simulink model "pack_96s"  (R2024b)
settings: Solver=ode4  StartTime=0.0  StopTime=T_stop  FixedStep=0.1  RelTol=1e-3
PreLoadFcn:
  | run(fullfile(fileparts(which('pack_96s')), '..', 'scripts', 'init_plant_model.m'));
undefined symbols (not defined in the file): cell_dSoC_pct, cell_Q_Ah, cell_RO_scale, cp_coolant, h_rad, I_bal_default, m_coolant, P_chiller_max, P_heater_max, T_cells_init, T_cool_off, T_cool_on, T_cool_target, T_heat_off, T_heat_on, T_heat_target, tau_chiller, tau_heater
settings Model: Creator=rayen  LastModifiedBy=dhia
settings DebuggingCC: AlgebraicLoopMsg=none

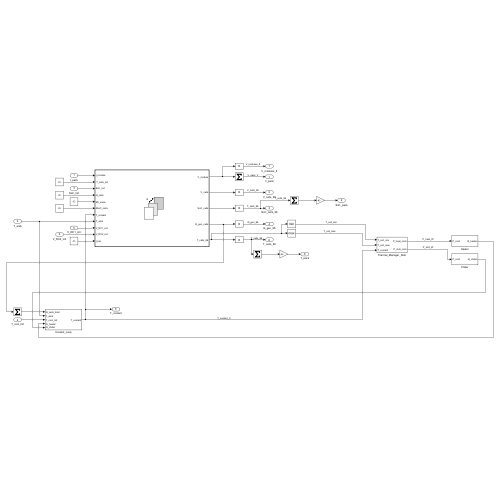
[thumbnail: Simulink's stored preview of the top-level diagram]
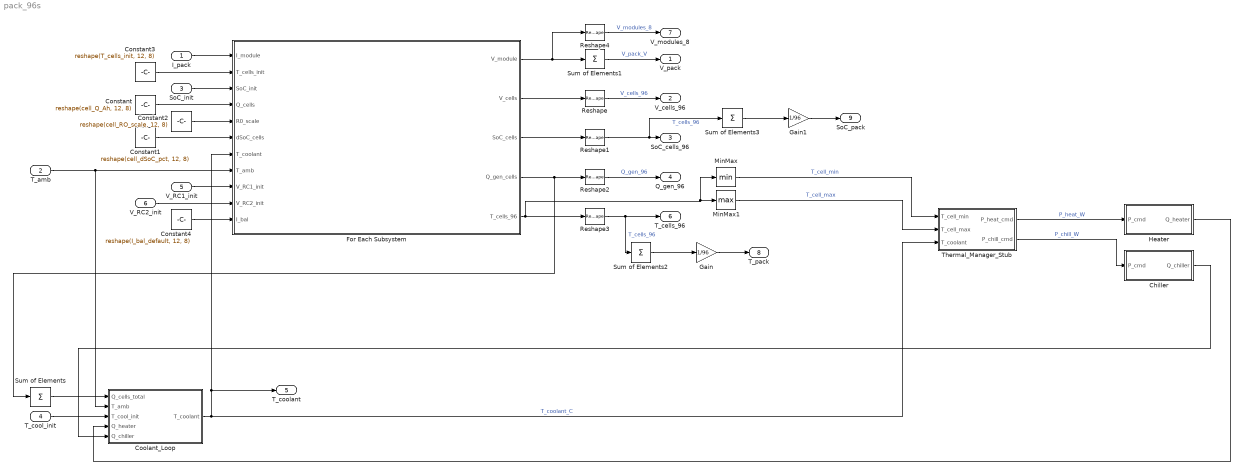
== system pack_96s ==
  I_pack : Inport
  T_amb : Inport  Port=2
  SoC_init : Inport  Port=3
  T_cool_init : Inport  Port=4
  V_RC1_init : Inport  Port=5
  V_RC2_init : Inport  Port=6
  Chiller : Subsystem
  Constant : Constant  Value=reshape(cell_Q_Ah, 12, 8)
  Constant1 : Constant  Value=reshape(cell_dSoC_pct, 12, 8)
  Constant2 : Constant  Value=reshape(cell_RO_scale, 12, 8)
  Constant3 : Constant  Value=reshape(T_cells_init, 12, 8)
  Constant4 : Constant  Value=reshape(I_bal_default, 12, 8)
  Coolant_Loop : Subsystem
  For Each Subsystem : Subsystem  TreatAsAtomicUnit=on
  Gain : Gain  Gain=1/96
  Gain1 : Gain  Gain=1/96
  Heater : Subsystem
  MinMax : MinMax
  MinMax1 : MinMax  Function=max
  Reshape{,1..3} (4 alike) : Reshape  OutputDimensionality=Customize  OutputDimensions=[96, 1]
  Reshape4 : Reshape  OutputDimensionality=Customize  OutputDimensions=[8, 1]
  Sum of Elements{,1..3} (4 alike) : Sum  Inputs=+
  Thermal_Manager_Stub : Subsystem
  V_pack : Outport
  V_cells_96 : Outport  Port=2
  SoC_cells_96 : Outport  Port=3
  Q_gen_96 : Outport  Port=4
  T_coolant : Outport  Port=5
  T_cells_96 : Outport  Port=6
  V_modules_8 : Outport  Port=7
  T_pack : Outport  Port=8
  SoC_pack : Outport  Port=9
  wires:
  I_pack/1 -> For Each Subsystem/1(I_module)
  SoC_init/1 -> For Each Subsystem/3(SoC_init)
  Constant/1 -> For Each Subsystem/4(Q_cells)
  Constant2/1 -> For Each Subsystem/5(R0_scale)
  Constant1/1 -> For Each Subsystem/6(dSoC_cells)
  For Each Subsystem/1(V_module) -> Reshape4/1, Sum of Elements1/1
  Sum of Elements1/1 -> V_pack/1  "V_pack_V"
  For Each Subsystem/2(V_cells) -> Reshape/1
  Reshape/1 -> V_cells_96/1  "V_cells_96"
  For Each Subsystem/3(SoC_cells) -> Reshape1/1
  Reshape2/1 -> Q_gen_96/1  "Q_gen_96"
  MinMax/1 -> Thermal_Manager_Stub/1(T_cell_min)  "T_cell_min"
  MinMax1/1 -> Thermal_Manager_Stub/2(T_cell_max)  "T_cell_max"
  For Each Subsystem/4(Q_gen_cells) -> Reshape2/1, Sum of Elements/1
  Sum of Elements/1 -> Coolant_Loop/1(Q_cells_total)
  Coolant_Loop/1(T_coolant) -> Thermal_Manager_Stub/3(T_coolant), T_coolant/1, For Each Subsystem/7(T_coolant)  "T_coolant_C"
  Thermal_Manager_Stub/1(P_heat_cmd) -> Heater/1(P_cmd)  "P_heat_W"
  Thermal_Manager_Stub/2(P_chill_cmd) -> Chiller/1(P_cmd)  "P_chill_W"
  Heater/1(Q_heater) -> Coolant_Loop/4(Q_heater)
  Chiller/1(Q_chiller) -> Coolant_Loop/5(Q_chiller)
  T_amb/1 -> Coolant_Loop/2(T_amb), For Each Subsystem/8(T_amb)
  For Each Subsystem/5(T_cells_96) -> MinMax/1, MinMax1/1, Reshape3/1
  T_cool_init/1 -> Coolant_Loop/3(T_cool_init)
  Constant3/1 -> For Each Subsystem/2(" T_cells_init")
  V_RC1_init/1 -> For Each Subsystem/9(V_RC1_init)
  V_RC2_init/1 -> For Each Subsystem/10(V_RC2_init)
  Reshape3/1 -> Sum of Elements2/1, T_cells_96/1  "T_cells_96"
  Constant4/1 -> For Each Subsystem/11(I_bal)
  Reshape4/1 -> V_modules_8/1  "V_modules_8"
  Sum of Elements2/1 -> Gain/1
  Gain/1 -> T_pack/1
  Reshape1/1 -> Sum of Elements3/1, SoC_cells_96/1  "T_cells_96"
  Sum of Elements3/1 -> Gain1/1
  Gain1/1 -> SoC_pack/1

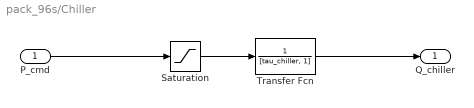
== system pack_96s/Chiller ==
  P_cmd : Inport
  Saturation : Saturate  UpperLimit=P_chiller_max  LowerLimit=0
  Transfer Fcn : TransferFcn  Denominator=[tau_chiller, 1]
  Q_chiller : Outport
  wires:
  Transfer Fcn/1 -> Q_chiller/1
  Saturation/1 -> Transfer Fcn/1
  P_cmd/1 -> Saturation/1

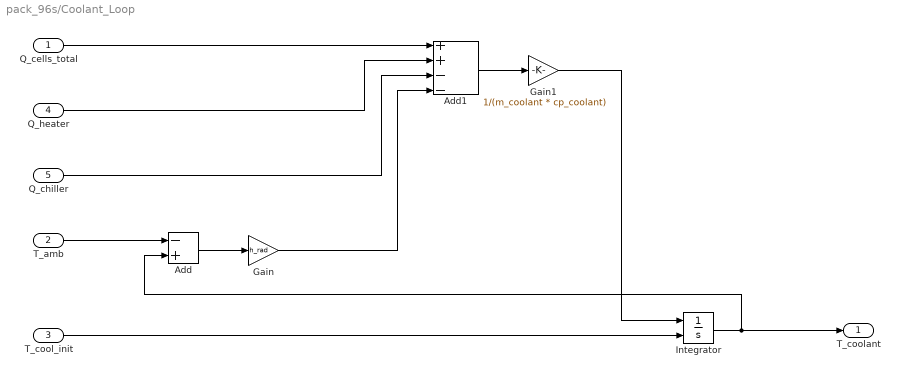
== system pack_96s/Coolant_Loop ==
  Q_cells_total : Inport
  T_amb : Inport  Port=2
  T_cool_init : Inport  Port=3
  Q_heater : Inport  Port=4
  Q_chiller : Inport  Port=5
  Add : Sum  Inputs=-+
  Add1 : Sum  Inputs=++--
  Gain : Gain  Gain=h_rad
  Gain1 : Gain  Gain=1/(m_coolant * cp_coolant)
  Integrator : Integrator  InitialConditionSource=external  LimitOutput=on  UpperSaturationLimit=80  LowerSaturationLimit=-40
  T_coolant : Outport
  wires:
  T_cool_init/1 -> Integrator/2
  Integrator/1 -> Add/2, T_coolant/1
  T_amb/1 -> Add/1
  Add/1 -> Gain/1
  Q_cells_total/1 -> Add1/1
  Q_heater/1 -> Add1/2
  Q_chiller/1 -> Add1/3
  Gain/1 -> Add1/4
  Add1/1 -> Gain1/1
  Gain1/1 -> Integrator/1

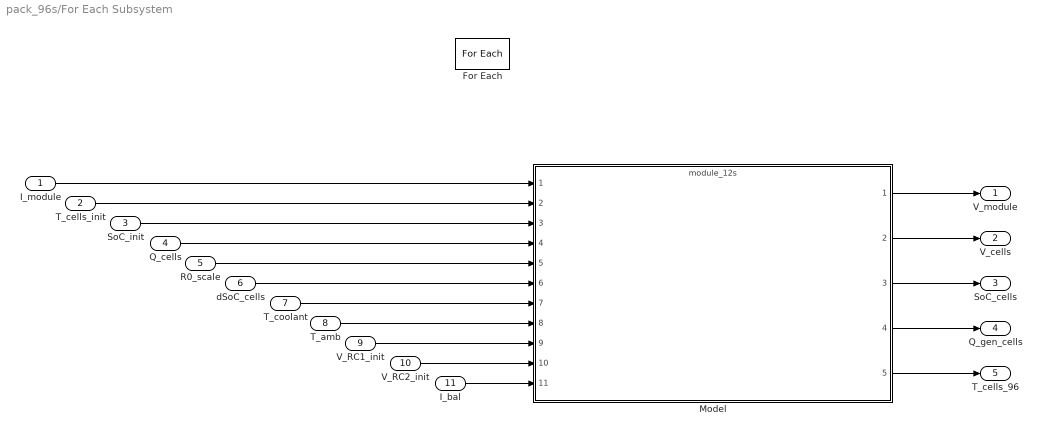
== system pack_96s/For Each Subsystem ==
  I_module : Inport
  " T_cells_init" : Inport  Port=2  Partition=on  PartitionDimension=2  PartitionWidth=1  PartitionOffset=0
  SoC_init : Inport  Port=3
  Q_cells : Inport  Port=4  Partition=on  PartitionDimension=2  PartitionWidth=1  PartitionOffset=0
  R0_scale : Inport  Port=5  Partition=on  PartitionDimension=2  PartitionWidth=1  PartitionOffset=0
  dSoC_cells : Inport  Port=6  Partition=on  PartitionDimension=2  PartitionWidth=1  PartitionOffset=0
  T_coolant : Inport  Port=7
  T_amb : Inport  Port=8
  V_RC1_init : Inport  Port=9
  V_RC2_init : Inport  Port=10
  I_bal : Inport  Port=11  Partition=on  PartitionDimension=2  PartitionWidth=1  PartitionOffset=0
  For Each : ForEach  DisableCoverage=on
  Model : ModelReference  ModelNameDialog=module_12s.slx  ModelReferenceVersion=1.30
  V_module : Outport  ConcatenationDimension=1
  V_cells : Outport  Port=2  ConcatenationDimension=1
  SoC_cells : Outport  Port=3  ConcatenationDimension=1
  Q_gen_cells : Outport  Port=4  ConcatenationDimension=1
  T_cells_96 : Outport  Port=5  ConcatenationDimension=1
  wires:
  I_module/1 -> Model/1
  Q_cells/1 -> Model/4
  SoC_init/1 -> Model/3
  " T_cells_init"/1 -> Model/2
  dSoC_cells/1 -> Model/6
  R0_scale/1 -> Model/5
  Model/4 -> Q_gen_cells/1
  Model/3 -> SoC_cells/1
  Model/2 -> V_cells/1
  Model/1 -> V_module/1
  Model/5 -> T_cells_96/1
  T_coolant/1 -> Model/7
  T_amb/1 -> Model/8
  V_RC2_init/1 -> Model/10
  V_RC1_init/1 -> Model/9
  I_bal/1 -> Model/11

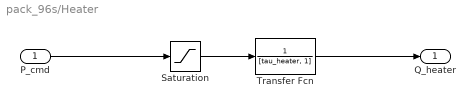
== system pack_96s/Heater ==
  P_cmd : Inport
  Saturation : Saturate  UpperLimit=P_heater_max  LowerLimit=0
  Transfer Fcn : TransferFcn  Denominator=[tau_heater, 1]
  Q_heater : Outport
  wires:
  P_cmd/1 -> Saturation/1
  Saturation/1 -> Transfer Fcn/1
  Transfer Fcn/1 -> Q_heater/1

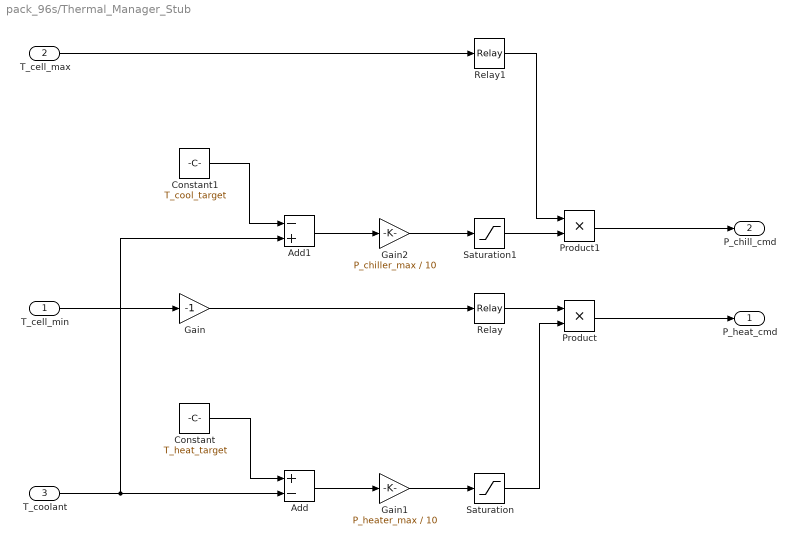
== system pack_96s/Thermal_Manager_Stub ==
  T_cell_min : Inport
  T_cell_max : Inport  Port=2
  T_coolant : Inport  Port=3
  Add : Sum  Inputs=+-
  Add1 : Sum  Inputs=-+
  Constant : Constant  Value=T_heat_target
  Constant1 : Constant  Value=T_cool_target
  Gain : Gain  Gain=-1
  Gain1 : Gain  Gain=P_heater_max / 10
  Gain2 : Gain  Gain=P_chiller_max / 10
  Product : Product
  Product1 : Product
  Relay : Relay  OnSwitchValue=-T_heat_on  OffSwitchValue=-T_heat_off
  Relay1 : Relay  OnSwitchValue=T_cool_on  OffSwitchValue=T_cool_off
  Saturation : Saturate  UpperLimit=P_heater_max  LowerLimit=0
  Saturation1 : Saturate  UpperLimit=P_chiller_max  LowerLimit=0
  P_heat_cmd : Outport
  P_chill_cmd : Outport  Port=2
  wires:
  T_coolant/1 -> Add1/2, Add/2
  Constant/1 -> Add/1
  Add/1 -> Gain1/1
  T_cell_min/1 -> Gain/1
  Product/1 -> P_heat_cmd/1
  Relay1/1 -> Product1/1
  Product1/1 -> P_chill_cmd/1
  Gain/1 -> Relay/1
  Relay/1 -> Product/1
  Saturation/1 -> Product/2
  Gain1/1 -> Saturation/1
  T_cell_max/1 -> Relay1/1
  Saturation1/1 -> Product1/2
  Gain2/1 -> Saturation1/1
  Add1/1 -> Gain2/1
  Constant1/1 -> Add1/1
